simulink model "beluga_model"  (R2016b)
settings: Solver=FixedStepAuto  StartTime=0.0  StopTime=10.0  FixedStep=0.01  RelTol=1e-3
values from neighbouring files (symbols this model uses):
  Ix = 0.05    [belugaSimulation.m]    (also in belugaStep.m; iverSimulation.m = 0; matlab.mat)
  Iy = 2.05    [belugaSimulation.m]    (also in belugaStep.m; iverSimulation.m = 0; matlab.mat)
  Iz = 2.06    [belugaSimulation.m]    (also in belugaStep.m; iverSimulation.m = 0; matlab.mat)
  K_pdot = -0.0704    [belugaSimulation.m]    (also in belugaStep.m; iverSimulation.m = 0; matlab.mat)
  m = 16.7/2.2    (= 7.59090909091)    [belugaSimulation.m]    (also in belugaStep.m = 4.2173; gps_state_est.m = 1; iverSimulation.m = 0; lin_test.m = 20.2)
  M_qdot = -3.2455    [belugaSimulation.m]    (also in belugaStep.m; iverSimulation.m = 0; matlab.mat)
  M_wdot = 2.5656    [belugaSimulation.m]    (also in belugaStep.m; iverSimulation.m = 0; matlab.mat)
  N_rdot = -3.2455    [belugaSimulation.m]    (also in belugaStep.m; iverSimulation.m = 0; matlab.mat)
  N_vdot = -2.5656    [belugaSimulation.m]    (also in belugaStep.m; iverSimulation.m = 0; matlab.mat)
  X_udot = -0.51334    [belugaSimulation.m]    (also in belugaStep.m; iverSimulation.m = 0; matlab.mat)
  xg = 0    [belugaSimulation.m]    (also in belugaStep.m; iverSimulation.m; matlab.mat)
  Y_rdot = -2.5656    [belugaSimulation.m]    (also in belugaStep.m; iverSimulation.m = 0; matlab.mat)
  Y_vdot = -23.8314    [belugaSimulation.m]    (also in belugaStep.m; iverSimulation.m = 0; matlab.mat)
  Z_qdot = 2.5656    [belugaSimulation.m]    (also in belugaStep.m; iverSimulation.m = 0; matlab.mat)
  Z_wdot = -23.8314    [belugaSimulation.m]    (also in belugaStep.m; iverSimulation.m = 0; matlab.mat)
  zg = 0    [belugaSimulation.m]    (also in belugaStep.m; iverSimulation.m; matlab.mat)
libraries: dspinverses x1
settings Model: Creator=HMCLoaner  LastModifiedBy=HMCLoaner

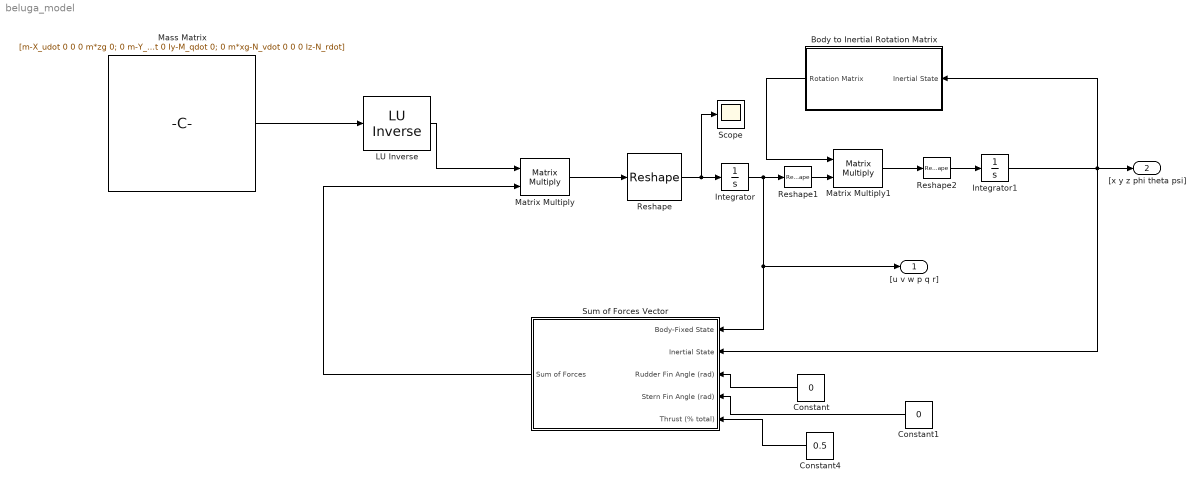
== system beluga_model ==
  " LU Inverse" : dspinverses/ LU Inverse
  Body to Inertial Rotation Matrix : Subsystem
  Constant : Constant  Value=0
  Constant1 : Constant  Value=0
  Constant4 : Constant  Value=0.5
  Integrator : Integrator  InitialCondition=[0 0 0 0 0 0]'
  Integrator1 : Integrator  InitialCondition=[0 0 0 0 0 0]'
  "Mass Matrix " : Constant  Value=[m-X_udot 0 0 0 m*zg 0; 0 m-Y_vdot 0 -m*zg 0 m*xg-Y_rdot; 0 0 m-Z_wdot 0 -m*xg-Z_qdot 0; 0 -m*zg 0 Ix-K_pdot 0 0; m*zg 0 -m*xg-M_wdot 0 Iy-M_qdot 0; 0 m*xg-N_vdot 0 0 0 Iz-N_rdot]  VectorParams1D=off
  Matrix Multiply : Product  Multiplication=Matrix(*)
  Matrix Multiply1 : Product  Multiplication=Matrix(*)
  Reshape : Reshape  OutputDimensions=3
  Reshape1 : Reshape  OutputDimensions=[1,6]
  Reshape2 : Reshape  OutputDimensions=[6,1]
  Scope : Scope
  Sum of Forces Vector : Subsystem
  "[u v w p q r]" : Outport
  "[x y z phi theta psi]" : Outport  Port=2
  wires:
  Reshape/1 -> Scope/1, Integrator/1
  Matrix Multiply/1 -> Reshape/1
  " LU Inverse"/1 -> Matrix Multiply/1
  Integrator/1 -> "[u v w p q r]"/1, Sum of Forces Vector/1(Body-Fixed State), Reshape1/1
  Reshape1/1 -> Matrix Multiply1/2
  Reshape2/1 -> Integrator1/1
  Matrix Multiply1/1 -> Reshape2/1
  "Mass Matrix "/1 -> " LU Inverse"/1
  Body to Inertial Rotation Matrix/1(Rotation Matrix) -> Matrix Multiply1/1
  Sum of Forces Vector/1(Sum of Forces) -> Matrix Multiply/2
  Constant/1 -> Sum of Forces Vector/3(Rudder Fin Angle (rad))
  Constant1/1 -> Sum of Forces Vector/4(Stern Fin Angle (rad))
  Integrator1/1 -> "[x y z phi theta psi]"/1, Sum of Forces Vector/2(Inertial State), Body to Inertial Rotation Matrix/1(Inertial State)
  Constant4/1 -> Sum of Forces Vector/5(Thrust (% total))

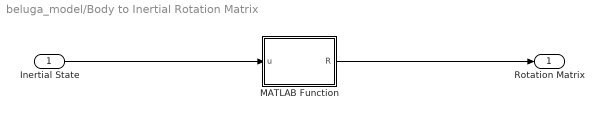
== system beluga_model/Body to Inertial Rotation Matrix ==
  Inertial State : Inport
  MATLAB Function : MATLAB Function  TreatAsAtomicUnit=on
  Rotation Matrix : Outport  PortDimensions=[6,6]
  wires:
  MATLAB Function/1(R) -> Rotation Matrix/1
  Inertial State/1 -> MATLAB Function/1(u)

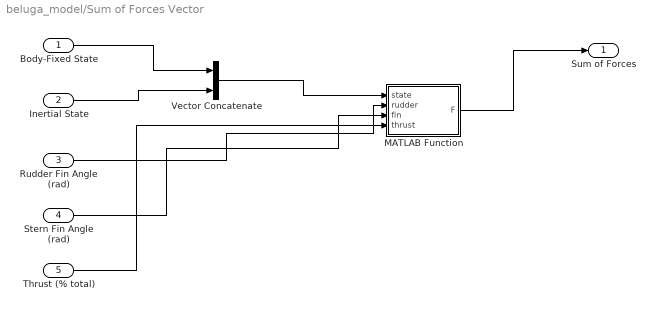
== system beluga_model/Sum of Forces Vector ==
  Body-Fixed State : Inport
  Inertial State : Inport  Port=2
  Rudder Fin Angle (rad) : Inport  Port=3
  Stern Fin Angle (rad) : Inport  Port=4
  Thrust (% total) : Inport  Port=5
  MATLAB Function : MATLAB Function  TreatAsAtomicUnit=on
  Vector Concatenate : Concatenate
  Sum of Forces : Outport
  wires:
  Body-Fixed State/1 -> Vector Concatenate/1
  Inertial State/1 -> Vector Concatenate/2
  Vector Concatenate/1 -> MATLAB Function/1(state)
  Rudder Fin Angle (rad)/1 -> MATLAB Function/2(rudder)
  Stern Fin Angle (rad)/1 -> MATLAB Function/3(fin)
  MATLAB Function/1(F) -> Sum of Forces/1
  Thrust (% total)/1 -> MATLAB Function/4(thrust)

== matlab function beluga_model/Sum of Forces Vector/MATLAB Function ==
  data: state input; F output; rudder input; fin input; thrust input
function F = fcn(state, rudder, fin, thrust)
    
    %% Constants
    %disp('Calc Nonlinear Coeffs')
    %Conversion Factors:
    i2m = 0.0254; %Conversion factor (inches to meters)
    lb2N = 4.44822162; %Conversion factor (lbs-force to Newtons)
    %Water Characteristics:
    %U = 1.5; %nominal velocity (m/s)
    U = 1; %2 knots
    rho = 1.03*10^(3); %seawater density (kg/m^3)
    %****Iver2 Hull Parameters*********************
    a = 8*i2m;
    a_offset = 0*i2m;
    b = 33.375*i2m;
    c = 7.34*i2m;
    c_offset = 1.04*i2m;
    d = 5.83*i2m;
    l = 47.67*i2m;
    Tail_angle = 35.5*pi/180;
    n = 2;
    %****************************************
    %**********Iver2 Moments of Inertia *****
    I_x = 0.05; %kg*m^2
    Iyy = 2.05; %kg*m^2
    Izz = 2.06; %kg*m^2
    %***************************************
    %Measured Parameters:
    W = 41.33*lb2N;
    m = W/9.8;
    B = 41.77*lb2N;
    %Measured or Estimated Centers of Buoyancy and Gravity
    xcg = 0*i2m;
    ycg = 0*i2m;
    zcg = 0.089*i2m;
    xcb = -23.72*i2m;
    ycb = 0*i2m;
    zcb = 0.03*i2m;
    %Vehicle parameters wrt. origin at the center of buoyancy
    x_g = 0;
    y_g = 0;
    z_g = 10*(zcg - zcb); %better COG-COB separation
    x_b = 0;
    y_b = 0;
    z_b = 0;
    %Fin characteristic parameters:
    fin1 = 2.54*i2m;
    fin2 = 1.92*i2m;
    fin3 = 5.7*i2m;
    fin4 = 1.26*i2m;
    fin5 = 3.51*i2m;
    fin6 = 4.5*i2m;
    %***********************Calculate The Non-Linear Coefficients**************
    %**************************************************************************
    %*****************************Axial Drag***********************************
    %Theoretical Drag Coeffecient: ( REMUS Eq 4.7)
    css = 3.397*10^(-3); %Schoenherr's value for flat plate skin friction
    Ap = l*d; %vehicle plan area
    Af = pi*(d/2)^2; %vehicle frontal area
    Cd = css*pi*Ap/Af*(1+60*(d/l)^3+0.0025*(l/d)); %drag coefficient estimate
    X_u_abs_u = -1/2*rho*Cd*Af; %Linear axial drag coefficient (kg/s)
    %*****************************Crossflow Drag*******************************
    %Define integration step size and limits of integration
    dx = 0.01; %integration step size
    %****Iver2 Values*****
    xn = abs(xcb)-(a-a_offset);
    xn2 = xn + (a-a_offset);
    xt2 = -(b-xn);
    xt = xt2 - (c - c_offset);
    xf = xt + fin4;
    xf2 = xt+fin6;
    lf = a+b-a_offset; %vehicle forward length
    %*********************
    Cdc = 1.1; %crossflow drag coefficient of a cylinder(Hoerner)
    taper = (fin5 - fin4)/(fin6 - fin4); %fin taper ratio
    Cdf = 0.1 + 0.7*taper; %control fin crossflow drag coefficient
    Sfin = 1/2*(fin1-fin2)*(fin6-fin4)+1/2*(fin6-fin5)*(fin3-fin1)+...
     (fin6-fin4)*(fin3-fin1); %control fin planform area
    xfin = xf2; %fin moment arm wrt origin at COB
    intg = cdrag(xt,xt2,xn,xn2,d,a,a_offset,n,c,Tail_angle,l,lf,dx,xcb);
    Z_w_abs_w = -1/2*rho*Cdc*intg - 2*(1/2*rho*Sfin*Cdf);
    Y_v_abs_v = Z_w_abs_w;
    intg = cdrag(xt,xt2,xn,xn2,d,a,a_offset,n,c,Tail_angle,l,lf,dx,xcb);
    M_w_abs_w = -1/2*rho*Cdc*intg - 2*xfin*(1/2*rho*Sfin*Cdf);
    N_v_abs_v = -M_w_abs_w;
    intg = cdrag(xt,xt2,xn,xn2,d,a,a_offset,n,c,Tail_angle,l,lf,dx,xcb);
    Zq_abs_q = 1/2*rho*Cdc*intg + 2*xfin*abs(xfin)*(1/2*rho*Sfin*Cdf);
    Y_r_abs_r = -Zq_abs_q;
    intg = cdrag(xt,xt2,xn,xn2,d,a,a_offset,n,c,Tail_angle,l,lf,dx,xcb);
    M_q_abs_q = -1/2*rho*Cdc*intg - 2*(xfin^3)*(1/2*rho*Sfin*Cdf);
    N_r_abs_r = M_q_abs_q;
    %Rolling Drag
    K_p_abs_p = -1.3*10^(-1); %Used REMUS VALUE
    %*****************************Added Mass***********************************
    %Define axial added mass parameters:
    alpha = 0.03585; %From table 4.1 of REMUS
    afin = fin3; %max fin height above the centerline
    %Calculate coefficients
    Xu_dot = -4*alpha*rho*pi/3*(l/2)*(d/2)^2;
    %intg = cdrag(xt,xf,xf2,xt2,xn,xn2,d,a,a_offset,n,c,l,lf,rho,afin,...
     %dx,Tail_angle,xcb);
    Yv_dot = intg;
    Zw_dot = Yv_dot;
    %intg = cdrag(xt,xf,xf2,xt2,xn,xn2,d,a,a_offset,n,c,l,lf,rho,afin,...
     %dx,Tail_angle,xcb);
    Mw_dot = intg; %Actual Equations in 4.20
    Nv_dot = -Mw_dot;
    Yr_dot = Nv_dot;
    Zq_dot = Mw_dot;
    %intg = cdrag(xt,xf,xf2,xt2,xn,xn2,d,a,a_offset,n,c,l,lf,rho,afin,...
     %dx,Tail_angle,xcb);
    Mq_dot = intg;
    Nr_dot = Mq_dot;
    %Rolling added mass:
    Kp_dot = -7.04*10^(-2); %kg*m^2/rad
    %Added mass cross-terms:
    X_wq = Zw_dot; %kg/rad
    X_qq = Zq_dot; %kg*m/rad
    X_vr = -Yv_dot; %kg/rad;
    X_rr = -Yr_dot; %kg*m/rad
    Yura = Xu_dot; %kg/rad
    Y_wp = -Zw_dot; %kg/rad
    Y_pq = -Zq_dot; %kg*m/rad
    Zuqa = -Xu_dot; %kg/rad
    Z_vp = Yv_dot; %kg/rad
    Z_rp = Yr_dot; %kg/rad
    Muwa = -(Zw_dot - Xu_dot); %kg
    M_vp = -Yr_dot; %kg*m/rad
    M_rp = (Kp_dot - Nr_dot); %kg*m^2/rad^2
    Muqa = -Zq_dot; %kg*m/rad
    Nuva = -(Xu_dot - Yv_dot); %kg
    N_wp = Zq_dot; %kg*m/rad
    N_pq = -(Kp_dot - Mq_dot); %kg*m^2/rad^2
    Nura = Yr_dot; %kg*m/rad
    %***************************Body Lift Force/Moment*************************
    cydb = (l/d)*0.003*180/pi;
    xcp = -0.65*l - xcb;
    Zuwl = -1/2*rho*d^2*cydb;
    Muwl = -1/2*rho*d^2*cydb*xcp;
    Yuvl = -1/2*rho*d^2*cydb;
    Nuvl = 1/2*rho*d^2*cydb*xcp;
    %**************************Fin Lift Force**********************************
    %Define Fin Lift coefficients
    SpanAve = 1/2*( (fin3-fin2)+(fin3-fin1) ); %avg span of one fin
    ARe = 2*(SpanAve^2)/Sfin; %Effective wing aspect ratio
    Cla = inv( 1/(2*0.9*pi) + 1/(pi*ARe) );
    Yuvf = -1/2*rho*Cla*Sfin; %kg/m
    Y_uudr = -Yuvf; %kg/(m*rad)
    Zuwf = -1/2*rho*Cla*Sfin; %kg/m
    Z_uuds = Zuwf; %kg/(m*rad)
    Zuqf = 1/2*rho*Cla*Sfin*xfin; %kg/rad
    Yurf = -Zuqf; %kg/rad
    Muwf = 1/2*rho*Cla*Sfin*xfin; %kg
    M_uuds = Muwf; %kg/rad
    Nuvf = -1/2*rho*Cla*Sfin*xfin; %kg
    N_uudr = -Nuvf; %kg/rad
    Nurf = -1/2*rho*Cla*Sfin*xfin^2;%kg*m/rad
    Muqf = Nurf; %kg*m/rad
    %**************************Define Propeller Coefficients*******************
    %Note: Decreasing Xprop lowers the steady state surge velocity
    Xprop = 1/2*3*(-2.37*X_u_abs_u); %REMUS VALUES
    Kprop = 1/2*-5.43*10^(-1); %REMUS VALUES
    X_prop = thrust*Xprop; %Fudge factor to slow vehicle from 1.5 to 1 m/s
    K_prop = thrust*Kprop;
    %*********************Combine Like Terms**********************************
    %The following equations combine the like terms as shown in Section 4.7 of
    %the Remus paper.
    Y_uv = Yuvl + Yuvf;
    Y_ur = Yura + Yurf;
    Z_uw = Zuwl + Zuwf;
    Z_uq = Zuqa + Zuqf;
    M_uw = Muwa + Muwl + Muwf;
    M_uq = Muqa + Muqf;
    N_uv = Nuva + Nuvl + Nuvf;
    N_ur = Nura + Nurf;

    
    %% States and calculations
    % defining states
    u = state(1);
    v = state(2);
    w = state(3);
    p = state(4);
    q = state(5);
    r = state(6);
    
    x = state(7);
    y = state(8);
    z = state(9);
    phi = state(10);
    theta = state(11);
    psi = state(12);
    
    % Hydrostatic forces
    X_hs = -(W-B)*sin(theta);
    Y_hs = (W-B)*sin(phi)*cos(theta);
    Z_hs = (W-B)*cos(phi)*cos(theta);
    K_hs = (ycg*W-ycb*B)*cos(theta)*cos(phi)-(zcg*W-zcb*B)*cos(theta)*sin(phi);
    M_hs = -(xcg*W-xcb*B)*cos(theta)*cos(phi)-(zcg*W-zcb*B)*sin(theta);
    N_hs = (xcg*W-xcb*B)*cos(theta)*sin(phi)-(ycg*W-ycb*B)*sin(theta);
    
    % Drag forces
    X_drag = X_u_abs_u*u*abs(u);
    Y_drag = Y_v_abs_v*v*abs(v);
    Z_drag = Z_w_abs_w*w*abs(w);
    K_drag = K_p_abs_p*p*abs(p);
    M_drag = M_w_abs_w*w*abs(w)+M_q_abs_q*q*(abs(q));
    N_drag = N_v_abs_v*v*abs(v)+N_r_abs_r*r*abs(r);
    
    % Lift forces TODO
    X_lift = X_wq*w*q+X_qq*q^2+X_vr*v*r+X_rr*r^2;
    Y_lift = Y_wp*w*p+Y_pq*q*p+Y_ur*u*r+Y_uv*u*v;
    Z_lift = Z_uq*u*q+Z_vp*v*p+Z_rp*r*p+Z_uw*u*w;
    K_lift = 0;
    M_lift = M_uq*u*q+M_vp*v*p+M_rp*r*p+M_uw*u*w;
    N_lift = N_ur*u*r+N_wp*w*p+N_pq*p*q+N_uv*u*v;
    
    % Added mass TODO
    
    % Control Forces
    X_c = X_prop;
    Y_c = Y_uudr*u^2*rudder;
    Z_c = Z_uuds*u^2*fin;
    K_c = K_prop;
    M_c = M_uuds*u^2*fin;
    N_c = N_uudr*u^2*rudder;
    
    % output force vector
    X = X_hs+X_c+X_drag+X_lift;
    Y = Y_hs+Y_c+Y_drag+Y_lift;
    Z = Z_hs+Z_c+Z_drag+Z_lift;
    K = K_hs+K_c+K_drag+K_lift;
    M = M_hs+M_c+M_drag+M_lift;
    N = N_hs+N_c+N_drag+N_lift;
    F = [X Y Z K M N]'; 
    %F = [1 0 0 0 0 0]';
end

function intg = cdrag(xt,xt2,xn,xn2,d,a,a_offset,n,c,theta,l,lf,dx,xb)
%This function performs the integration for the first equation of 4.8 in
%the REMUS thesis
intg = 0;
xti = l;
for x = xt:dx:xt2
 %Need to adjust for the difference in origin definitions between the
 %radius functions and the body-coord with the following transform:
 Rx = ( 1/2*d - ( 3*d/(2*c^2) - tan(theta)/c )*(xti-lf)^2 + ...
 ( d/(c^3) - tan(theta)/(c^2) )*(xti - lf)^3 );
 xti = xti-dx;

 intg = intg + 2*Rx*dx;
end
for x = xt2:dx:xn
 Rx = d/2;
 intg = intg + 2*Rx*dx;
end
for x = xn:dx:xn2
 %Need to adjust for the difference in origin definitions betwee the
 %radius functions and the body-coord with the following transform:
 xi = -( x - abs(xb) + (a-a_offset) ) + a;
 Rx = ( 1/2*d*( 1 - ( (xi + a_offset-a)/a )^2 )^(1/n) );

 intg = intg + 2*Rx*dx;
end
end
%End of cdrag function

== matlab function beluga_model/Body to Inertial Rotation Matrix/MATLAB Function ==
  data: u input; R output
function R = fcn(u)
    % Inputs
    x = u(1);
    y = u(2);
    z = u(3);
    phi = u(4);
    theta = u(5);
    psi = u(6);
    
    % transformation
    cosphi = cos(phi);
    sinphi = sin(phi);
    costheta = cos(theta);
    sintheta = sin(theta);
    cospsi = cos(psi);
    sinpsi = sin(psi);

    R = zeros(6,6);
    R(1,1) = cospsi.*cosphi-costheta.*sinphi.*sinpsi;
    R(1,2) = sinphi.*cospsi+costheta.*cosphi.*sinpsi;
    R(1,3) = sintheta.*sinpsi;

    R(2,1) = -cosphi.*sinpsi-costheta.*cospsi.*sinphi;
    R(2,2) = -sinpsi.*sinphi+costheta.*cosphi.*cospsi;
    R(2,3) = sintheta.*cospsi;

    R(3,1) = sinphi.*sintheta;
    R(3,2) = -cosphi.*sintheta;
    R(3,3) = costheta;
    
    R(4,4) = 1;
    R(5,5) = 1;
    R(6,6) = 1;
end
